simulink model "aula2108"  (Simulink 7.1)
settings: Solver=ode45  StartTime=0.0  StopTime=30.0  RelTol=1e-3
settings Model: Creator=nu3_lab7  LastModifiedBy=nu3_lab7

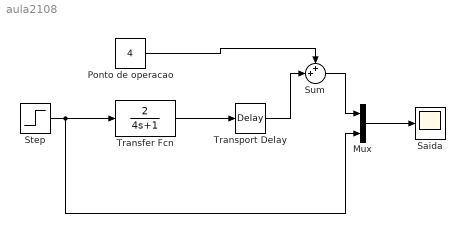
== system aula2108 ==
  Mux : Mux  Inputs=2
  Ponto de operacao : Constant  Value=4  OutDataType=sfix(16)  OutScaling=2^0
  Saida : Scope
  Step : Step  Time=0.1  After=3  SampleTime=0
  Sum : Sum  Inputs=++|  OutDataType=sfix(16)  OutScaling=2^0
  Transfer Fcn : TransferFcn  Numerator=[2]  Denominator=[4 1]
  Transport Delay : TransportDelay  DelayTime=3
  wires:
  Transport Delay/1 -> Sum/2
  Transfer Fcn/1 -> Transport Delay/1
  Ponto de operacao/1 -> Sum/1
  Step/1 -> Transfer Fcn/1, Mux/2
  Sum/1 -> Mux/1
  Mux/1 -> Saida/1
